simulink model "admittance_controller_test"  (R2025b)
settings: Solver=ode1  StartTime=0.0  StopTime=100  FixedStep=1/500.  RelTol=1e-3
libraries: sdu_controllers x1
settings Model: Creator=eld  LastModifiedBy=madla

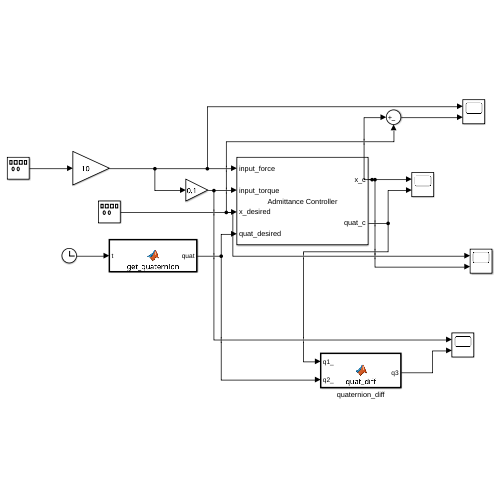
[thumbnail: Simulink's stored preview of the top-level diagram]
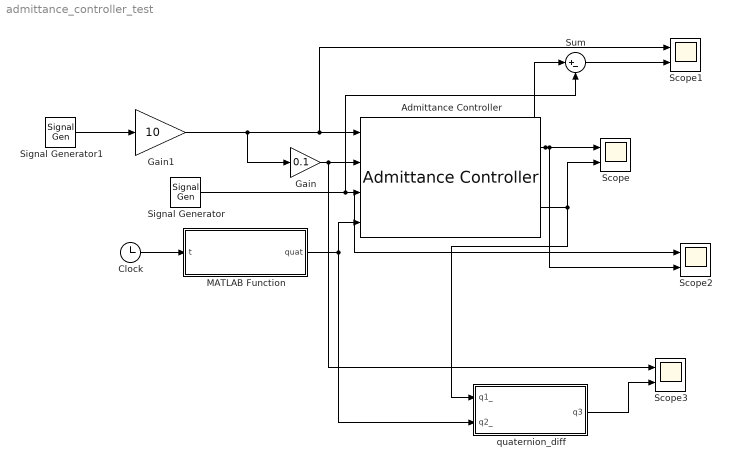
== system admittance_controller_test ==
  Admittance Controller : sdu_controllers/Controllers/Admittance Controller  Mp=eye( 3 )  Kp=eye( 3 )  Dp=eye( 3 )  Mo=eye( 3 )  Ko=eye( 3 )  Do=eye( 3 )  sample_time=1 / 500.  SimulateUsing=Interpreted execution
      settings: SourceProductName=SDU Controllers
  Clock : Clock
  Gain : Gain  Gain=0.1
  Gain1 : Gain  Gain=10
  MATLAB Function : MATLAB Function  TreatAsAtomicUnit=on
  Scope{,1..3} (4 alike) : Scope  NumInputPorts=2
      Scope settings: ActiveDisplayYMinimum=-52.908855833797759  ActiveDisplayYMaximum=52.908828332847349
      Scope1 settings: ActiveDisplayYMinimum=-37.5  ActiveDisplayYMaximum=37.5
      Scope2 settings: ActiveDisplayYMinimum=-3.7499999948138449  ActiveDisplayYMaximum=3.7499999988615755  DataLoggingVariableName=ScopeData2
      Scope3 settings: ActiveDisplayYMinimum=-3.75  ActiveDisplayYMaximum=3.75  DataLoggingVariableName=ScopeData3
  Signal Generator : SignalGenerator  Amplitude=[1, 2, 3]  Units=rad/sec
  Signal Generator1 : SignalGenerator  WaveForm=square  Amplitude=[1, 2, 3]  Frequency=[1.0,1.1,1.2] * 0.5  Units=rad/sec
  Sum : Sum  Inputs=|+-
  quaternion_diff : MATLAB Function  TreatAsAtomicUnit=on
  wires:
  Signal Generator/1 -> Admittance Controller/3, Scope2/1, Sum/2
  MATLAB Function/1(quat) -> Admittance Controller/4, quaternion_diff/2(q2_)
  Clock/1 -> MATLAB Function/1(t)
  Signal Generator1/1 -> Gain1/1
  Gain/1 -> Admittance Controller/2, Scope3/1
  Admittance Controller/1 -> Sum/1, Scope2/2, Scope/1
  Admittance Controller/2 -> Scope/2, quaternion_diff/1(q1_)
  Gain1/1 -> Gain/1, Admittance Controller/1, Scope1/1
  Sum/1 -> Scope1/2
  quaternion_diff/1(q3) -> Scope3/2

== matlab function admittance_controller_test/MATLAB Function ==
  data: t input; quat output
function quat = get_quaternion(t)

q1 = quaternion(1, 0, 0, 0);
q1 = q1 / norm(q1);

%
q2 = quaternion(2, 3, 4, 5);
q2 = q2 / norm(q2);

qout = slerp(q1, q2, t/100);

quat = compact(qout);

== matlab function admittance_controller_test/quaternion_diff ==
  data: q1_ input; q3 output; q2_ input
function q3 = quat_diff(q1_, q2_)

q1 = quaternion(q1_);
q2 = quaternion(q2_);

q3 = compact(q1 - q2);
